simulink model "gsm"  (R2015b)
settings: Solver=VariableStepDiscrete  StartTime=0.0  StopTime=inf  RelTol=1e-3
libraries: dspsigops x34, commblkintrlv2 x4, commdigbbndcpm2 x3, commcrc2 x2, commcnvcod2 x2, commsrccod2 x2, commrandsrc3 x1, commsink2 x1, commchan3 x1
(part 2 of 2)

== matlab function gsm/background5/background5/Data Burst/Subsystem3/Training Bits4 ==
  data: u input; y output
function y = fcn(u)
% This block supports an embeddable subset of the MATLAB language.
% See the help menu for details. 

training4 = [0,1,0,0,0,1,1,1,1,0,1,1,0,1,0,0,0,1,0,0,0,1,1,1,1,0];
y = training4;

== matlab function gsm/background5/background5/Data Burst/Subsystem4/Training Bits4 ==
  data: u input; y output
function y = fcn(u)
% This block supports an embeddable subset of the MATLAB language.
% See the help menu for details. 

training4 = [0,1,0,0,0,1,1,1,1,0,1,1,0,1,0,0,0,1,0,0,0,1,1,1,1,0];
y = training4;

== matlab function gsm/background5/background5/Data Burst/Subsystem5/Training Bits4 ==
  data: u input; y output
function y = fcn(u)
% This block supports an embeddable subset of the MATLAB language.
% See the help menu for details. 

training4 = [0,1,0,0,0,1,1,1,1,0,1,1,0,1,0,0,0,1,0,0,0,1,1,1,1,0];
y = training4;

== matlab function gsm/background5/background5/Data Burst/Subsystem6/Training Bits4 ==
  data: u input; y output
function y = fcn(u)
% This block supports an embeddable subset of the MATLAB language.
% See the help menu for details. 

training4 = [0,1,0,0,0,1,1,1,1,0,1,1,0,1,0,0,0,1,0,0,0,1,1,1,1,0];
y = training4;

== matlab function gsm/background5/background5/Data Burst/Subsystem7/Training Bits4 ==
  data: u input; y output
function y = fcn(u)
% This block supports an embeddable subset of the MATLAB language.
% See the help menu for details. 

training4 = [0,1,0,0,0,1,1,1,1,0,1,1,0,1,0,0,0,1,0,0,0,1,1,1,1,0];
y = training4;
